simulink library "sm_car_lib"  (R2024a)
settings: Solver=VariableStepAuto  StartTime=0.0  StopTime=10.0  RelTol=1e-3
undefined symbols (not defined in the file or in its folder): acc_theta, accel_ramp_rate, circ_out, clr_upr, Control, hp1, hp2, hp3, hp_in_f_ua, hp_in_r_ua, hp_la_out, hp_ua_out, Init, Newton, opc_upr, radius_upr, Raphson, RDF_Rough_Road, rhs_hp, Scene, ShaftF, ShaftR, Vehicle, Visual, X, Y, Z
libraries: sm_lib x117, $bdroot x97, nesl_utility x36, simulink x17, fl_lib x6, sharedtransformsys x3, Brakes_Elements x2, Driver_Gamepad_Xbox x2, Multibody_Parts_Lib x2, sm_car_scene_track_mallory_park_obstacle x2, Testrig_4Post_Inputs x2, Aero_Coefficients x1
(part 7 of 7)

== system sm_car_lib/Environment/CarWorldConfig/Mechanism Configuration/Constant Gravity ==
  MechanismConfiguration : sm_lib/Utilities/Mechanism Configuration  UniformGravity=Constant  GravityVector=GravityVector  GravityVectorUnits=m/s^2  LinearizationDelta=0.001  JointModeTransitionNonlinearIterations=2
  C : PMIOPort  Side=Right
  connections:
  MechanismConfiguration/RConn1 -- C/RConn1

== system sm_car_lib/Environment/CarWorldConfig/Mechanism Configuration/Variable GravityXY ==
  Constant : Constant  Value=acc_theta
  Constant1 : Constant  Value=GravityVector(3)
  MechanismConfiguration : sm_lib/Utilities/Mechanism Configuration  UniformGravity=TimeVarying  GravityVector=[0 0 -9.80665]  GravityVectorUnits=m/s^2  LinearizationDelta=0.001  JointModeTransitionNonlinearIterations=2
  Mux : Mux  Inputs=3
  Product : Product
  Product1 : Product
  Ramp1 : simulink/Sources/Ramp  slope=accel_ramp_rate  start=2  InitialOutput=0
  Scope : Scope
  Simulink-PS Converter : nesl_utility/Simulink-PS Converter  PhysicalDomain=network_engine_domain  SubClassName=ps_input  LeftPortType=input  RightPortType=output  PseudoPeriodic=off  Frequencies=[]  NoiseDistribution=none  NoiseParameters=[]  Unit=m/s^2  AffineConversion=off  FilteringAndDerivatives=provide  SimscapeFilterOrder=1  InputFilterTimeConstant=0.001  UdotUserProvided=0
  Sin : Trigonometry
  Sin1 : Trigonometry  Operator=cos
  C : PMIOPort  Side=Right
  wires:
  Ramp1/1 -> Product/2, Product1/2, Scope/1  "accel_xy"
  Product1/1 -> Mux/1
  Constant1/1 -> Mux/3
  Sin/1 -> Product/1
  Mux/1 -> Simulink-PS Converter/1
  Sin1/1 -> Product1/1
  Constant/1 -> Sin/1, Sin1/1
  Product/1 -> Mux/2
  connections:
  MechanismConfiguration/LConn1 -- Simulink-PS Converter/RConn1
  MechanismConfiguration/RConn1 -- C/RConn1

== system sm_car_lib/Inputs/Control Bus/Torque Input/Torque Front ==
  Gain : Gain
  Rate Limiter : RateLimiter  RisingSlewLimit=300  FallingSlewLimit=-300  SampleTimeMode=inherited
  Step Height : Gain  Gain=torque_value
  Step Off : Step  Time=off_time  After=-1  SampleTime=0  ZeroCross=off
  Step On : Step  Time=on_time  SampleTime=0  ZeroCross=off
  Sum : Sum  Inputs=|++
  MMotorRDemand : Outport  VectorParamsAs1DForOutWhenUnconnected=off
  wires:
  Gain/1 -> MMotorRDemand/1  "MMotorRDemand"
  Step Off/1 -> Sum/2
  Sum/1 -> Step Height/1
  Step On/1 -> Sum/1
  Rate Limiter/1 -> Gain/1
  Step Height/1 -> Rate Limiter/1

== system sm_car_lib/Inputs/Control Bus/Torque Input/Torque Rear ==
  Gain : Gain
  Rate Limiter : RateLimiter  RisingSlewLimit=300  FallingSlewLimit=-300  SampleTimeMode=inherited
  Step Height : Gain  Gain=torque_value
  Step Off : Step  Time=off_time  After=-1  SampleTime=0  ZeroCross=off
  Step On : Step  Time=on_time  SampleTime=0  ZeroCross=off
  Sum : Sum  Inputs=|++
  MMotorRDemand : Outport  VectorParamsAs1DForOutWhenUnconnected=off
  wires:
  Step Height/1 -> Rate Limiter/1
  Rate Limiter/1 -> Gain/1
  Step On/1 -> Sum/1
  Sum/1 -> Step Height/1
  Step Off/1 -> Sum/2
  Gain/1 -> MMotorRDemand/1  "MMotorRDemand"

== system sm_car_lib/Inputs/Control Bus Axle3/Torque Input/Torque Front ==
  Gain : Gain
  Rate Limiter : RateLimiter  RisingSlewLimit=300  FallingSlewLimit=-300  SampleTimeMode=inherited
  Step Height : Gain  Gain=torque_value
  Step Off : Step  Time=off_time  After=-1  SampleTime=0  ZeroCross=off
  Step On : Step  Time=on_time  SampleTime=0  ZeroCross=off
  Sum : Sum  Inputs=|++
  MMotorRDemand : Outport  VectorParamsAs1DForOutWhenUnconnected=off
  wires:
  Step Height/1 -> Rate Limiter/1
  Rate Limiter/1 -> Gain/1
  Step On/1 -> Sum/1
  Sum/1 -> Step Height/1
  Step Off/1 -> Sum/2
  Gain/1 -> MMotorRDemand/1  "MMotorRDemand"

== system sm_car_lib/Inputs/Control Bus Axle3/Torque Input/Torque Rear ==
  Gain : Gain
  Rate Limiter : RateLimiter  RisingSlewLimit=300  FallingSlewLimit=-300  SampleTimeMode=inherited
  Step Height : Gain  Gain=torque_value
  Step Off : Step  Time=off_time  After=-1  SampleTime=0  ZeroCross=off
  Step On : Step  Time=on_time  SampleTime=0  ZeroCross=off
  Sum : Sum  Inputs=|++
  MMotorRDemand : Outport  VectorParamsAs1DForOutWhenUnconnected=off
  wires:
  Gain/1 -> MMotorRDemand/1  "MMotorRDemand"
  Step Off/1 -> Sum/2
  Sum/1 -> Step Height/1
  Step On/1 -> Sum/1
  Rate Limiter/1 -> Gain/1
  Step Height/1 -> Rate Limiter/1

== system sm_car_lib/Inputs/DrvBus/Torque Input/Torque Front ==
  Gain : Gain  Gain=rPedalValue
  Step Off : Step  Time=off_time  After=-1  SampleTime=0  ZeroCross=off
  Step On : Step  Time=on_time  SampleTime=0  ZeroCross=off
  Sum : Sum  Inputs=|++
  rAccelPedal : Outport  VectorParamsAs1DForOutWhenUnconnected=off
  wires:
  Sum/1 -> Gain/1
  Step Off/1 -> Sum/2
  Step On/1 -> Sum/1
  Gain/1 -> rAccelPedal/1  "rAccelPedal"

== system sm_car_lib/Outputs/VehBus/Brakes/Subsystem ==
  Bus Creator : BusCreator  Inputs=2
  Constant : Constant
  Constant1 : Constant
  Whl : Outport  VectorParamsAs1DForOutWhenUnconnected=off
  wires:
  Constant/1 -> Bus Creator/1  "trq"
  Bus Creator/1 -> Whl/1
  Constant1/1 -> Bus Creator/2  "p"

== system sm_car_lib/Outputs/VehBus/Subsystem/Aero ==
  Bus Creator : BusCreator  Inputs=2
  Constant1 : Constant
  Constant3 : Constant
  Aero : Outport  VectorParamsAs1DForOutWhenUnconnected=off
  wires:
  Constant3/1 -> Bus Creator/1  "Fx"
  Constant1/1 -> Bus Creator/2  "Fz"
  Bus Creator/1 -> Aero/1  "Aero"

== system sm_car_lib/Outputs/VehBus/Subsystem/Damper ==
  Bus Creator5 : BusCreator  Inputs=4
  Subsystem : Subsystem
  Subsystem1 : $bdroot/Outputs/VehBus/Subsystem/Damper/Subsystem  SystemSampleTime=-1  VariantActivationTime=update diagram  AllowFlexibleInterface=on  Latency=0  AutoFrameSizeCalculation=off
  Subsystem2 : $bdroot/Outputs/VehBus/Subsystem/Damper/Subsystem  SystemSampleTime=-1  VariantActivationTime=update diagram  AllowFlexibleInterface=on  Latency=0  AutoFrameSizeCalculation=off
  Subsystem3 : $bdroot/Outputs/VehBus/Subsystem/Damper/Subsystem  SystemSampleTime=-1  VariantActivationTime=update diagram  AllowFlexibleInterface=on  Latency=0  AutoFrameSizeCalculation=off
  Damper : Outport  VectorParamsAs1DForOutWhenUnconnected=off
  wires:
  Subsystem3/1 -> Bus Creator5/4  "R2"
  Subsystem1/1 -> Bus Creator5/2  "R1"
  Bus Creator5/1 -> Damper/1  "Damper"
  Subsystem2/1 -> Bus Creator5/3  "L2"
  Subsystem/1(out) -> Bus Creator5/1  "L1"

== system sm_car_lib/Outputs/VehBus/Subsystem/Source ==
  Bus Creator : BusCreator  Inputs=15
  Constant1 : Constant  Value=[1 1 1]
  Constant{2..5,7..15} (13 alike) : Constant
  Constant6 : Constant  Value=[1 1 1]
  Whl : Outport  VectorParamsAs1DForOutWhenUnconnected=off
  wires:
  Constant11/1 -> Bus Creator/3  "n"
  Constant12/1 -> Bus Creator/4  "Fx"
  Constant1/1 -> Bus Creator/2  "xyz"
  Constant6/1 -> Bus Creator/1  "qxyz"
  Bus Creator/1 -> Whl/1
  Constant2/1 -> Bus Creator/5  "Fy"
  Constant3/1 -> Bus Creator/6  "Fz"
  Constant4/1 -> Bus Creator/7  "Mx"
  Constant5/1 -> Bus Creator/8  "My"
  Constant7/1 -> Bus Creator/9  "Mz"
  Constant8/1 -> Bus Creator/10  "rSlip"
  Constant9/1 -> Bus Creator/11  "aSlip"
  Constant10/1 -> Bus Creator/12  "aCamber"
  Constant13/1 -> Bus Creator/13  "vx"
  Constant14/1 -> Bus Creator/14  "rMuX"
  Constant15/1 -> Bus Creator/15  "rMuY"

== system sm_car_lib/Outputs/VehBus/Subsystem/Spring ==
  Bus Creator5 : BusCreator  Inputs=4
  Source : Subsystem
  Subsystem1 : $bdroot/Outputs/VehBus/Subsystem/Spring/Source  SystemSampleTime=-1  VariantActivationTime=update diagram  AllowFlexibleInterface=on  Latency=0  AutoFrameSizeCalculation=off
  Subsystem2 : $bdroot/Outputs/VehBus/Subsystem/Spring/Source  SystemSampleTime=-1  VariantActivationTime=update diagram  AllowFlexibleInterface=on  Latency=0  AutoFrameSizeCalculation=off
  Subsystem3 : $bdroot/Outputs/VehBus/Subsystem/Spring/Source  SystemSampleTime=-1  VariantActivationTime=update diagram  AllowFlexibleInterface=on  Latency=0  AutoFrameSizeCalculation=off
  Spring : Outport  VectorParamsAs1DForOutWhenUnconnected=off
  wires:
  Bus Creator5/1 -> Spring/1  "Spring"
  Subsystem1/1 -> Bus Creator5/2  "R1"
  Subsystem2/1 -> Bus Creator5/3  "L2"
  Subsystem3/1 -> Bus Creator5/4  "R2"
  Source/1(out) -> Bus Creator5/1  "L1"

== system sm_car_lib/Sensors/Body Sensor/Roll Pitch/Calculate aPitch ==
  Roll Angle : Inport
  uvec : Inport  Port=2
  Asin : Trigonometry  Operator=asin
  Cos : Trigonometry  Operator=cos
  Divide : Product  Inputs=*/
  Divide1 : Product  Inputs=*/
  Selector : Selector  InputPortWidth=3  IndexOptions=Index vector (dialog)  Indices=[3]  OutputSizes=1
  magnitude : Fcn  Expr=sqrt(u(1)*u(1)+u(2)*u(2)+u(3)*u(3))
  Angle : Outport  VectorParamsAs1DForOutWhenUnconnected=off
  wires:
  Divide1/1 -> Asin/1
  uvec/1 -> magnitude/1, Selector/1
  magnitude/1 -> Divide1/2
  Selector/1 -> Divide/1
  Roll Angle/1 -> Cos/1
  Asin/1 -> Angle/1
  Divide/1 -> Divide1/1
  Cos/1 -> Divide/2

== system sm_car_lib/Sensors/Body Sensor/Roll Pitch/Calculate aRoll ==
  uvec : Inport
  Demux : Demux  Outputs=3
  Mux : Mux  Inputs=2
  Trigonometric Function1 : Trigonometry  Operator=atan2
  magnitude : Fcn  Expr=sqrt(u(1)*u(1)+u(2)*u(2))
  Angle : Outport  VectorParamsAs1DForOutWhenUnconnected=off
  wires:
  Demux/2 -> Mux/2
  magnitude/1 -> Trigonometric Function1/2
  Mux/1 -> magnitude/1
  Demux/3 -> Trigonometric Function1/1
  Trigonometric Function1/1 -> Angle/1
  uvec/1 -> Demux/1
  Demux/1 -> Mux/1

== system sm_car_lib/Utilities/Q to Z-Y-X Extrinsic/Subsystem/Subsystem ==
  In : Inport
  If : If  IfExpression=u1 > 1  ElseIfExpressions=u1 < -1
  If Action Subsystem : sharedtransformsys/Protect asincos input/If Action Subsystem  SystemSampleTime=-1  VariantActivationTime=update diagram  AllowFlexibleInterface=on  Latency=0  AutoFrameSizeCalculation=off
  If Action Subsystem1 : sharedtransformsys/Protect asincos input/If Action Subsystem1  SystemSampleTime=-1  VariantActivationTime=update diagram  AllowFlexibleInterface=on  Latency=0  AutoFrameSizeCalculation=off
  If Action Subsystem2 : sharedtransformsys/Protect asincos input/If Action Subsystem2  SystemSampleTime=-1  VariantActivationTime=update diagram  AllowFlexibleInterface=on  Latency=0  AutoFrameSizeCalculation=off
  Merge : Merge  Inputs=3
  Out : Outport  VectorParamsAs1DForOutWhenUnconnected=off
  wires:
  If Action Subsystem1/1 -> Merge/2
  If/1 -> If Action Subsystem/Action
  In/1 -> If/1, If Action Subsystem2/1
  If/3 -> If Action Subsystem2/Action
  If Action Subsystem2/1 -> Merge/3
  If/2 -> If Action Subsystem1/Action
  If Action Subsystem/1 -> Merge/1
  Merge/1 -> Out/1

== system sm_car_lib/Utilities/Q to Z-Y-X Extrinsic/Subsystem1/Subsystem ==
  In1 : Inport
  Demux : Demux
  Product{,1..3} (4 alike) : Product
  Sum : Sum  Inputs=4
  sqrt : Sqrt  AlgorithmType=Newton-Raphson
  Out1 : Outport  VectorParamsAs1DForOutWhenUnconnected=off
  wires:
  Sum/1 -> sqrt/1
  sqrt/1 -> Out1/1
  In1/1 -> Demux/1
  Product3/1 -> Sum/4
  Demux/2 -> Product1/1, Product1/2
  Demux/1 -> Product/1, Product/2
  Product2/1 -> Sum/3
  Product/1 -> Sum/1
  Demux/3 -> Product2/1, Product2/2
  Product1/1 -> Sum/2
  Demux/4 -> Product3/1, Product3/2

== system sm_car_lib/Control/Brake Control/ABS/Sensor/missing tooth ==
  <omega> : Inport
  <qxyz> : Inport  Port=2
  Constant : Constant  Value=2*pi
  Constant1 : Constant  Value=0.5
  Constant2 : Constant
  Product : Product
  Rem : Math  Operator=rem  SignedPower=on
  Scope : Scope  NumInputPorts=5
  Selector : Selector  InputPortWidth=3  IndexOptions=Index vector (dialog)  Indices=[2]  OutputSizes=1
  Subsystem : Subsystem  mask{int_limit_upper=25/48*2*pi, int_limit_lower=22/48*2*pi}
      mask prompts: int_limit_upper "Upper Limit"; int_limit_lower "Lower Limit"
      mask TypeOptions int_limit_upper: Upper Limit/Value
      mask TypeOptions int_limit_lower: Lower Limit/Value
  Switch : Switch  Criteria=u2 > Threshold  Threshold=0.5  SaturateOnIntegerOverflow=off  InputSameDT=off
  Out1 : Outport  VectorParamsAs1DForOutWhenUnconnected=off
  wires:
  <qxyz>/1 -> Scope/1, Selector/1
  Constant/1 -> Rem/2
  Rem/1 -> Scope/3, Subsystem/1(u)
  Selector/1 -> Scope/2, Rem/1
  Subsystem/1(y) -> Scope/4, Switch/2
  Switch/1 -> Scope/5, Product/2
  Constant1/1 -> Switch/1
  Constant2/1 -> Switch/3
  <omega>/1 -> Product/1
  Product/1 -> Out1/1

== system sm_car_lib/Outputs/VehBus/Subsystem/Damper/Subsystem ==
  Bus Creator : BusCreator  Inputs=4
  Constant{1..4} (4 alike) : Constant
  out : Outport  VectorParamsAs1DForOutWhenUnconnected=off
  wires:
  Constant2/1 -> Bus Creator/3  "xDamper"
  Bus Creator/1 -> out/1
  Constant3/1 -> Bus Creator/4  "vDamper"
  Constant1/1 -> Bus Creator/2  "FBumpstop"
  Constant4/1 -> Bus Creator/1  "FDamper"

== system sm_car_lib/Outputs/VehBus/Subsystem/Spring/Source ==
  Bus Creator : BusCreator  Inputs=2
  Constant1 : Constant
  Constant4 : Constant
  out : Outport  VectorParamsAs1DForOutWhenUnconnected=off
  wires:
  Constant1/1 -> Bus Creator/2  "FSpring"
  Constant4/1 -> Bus Creator/1  "xSpring"
  Bus Creator/1 -> out/1

== system sm_car_lib/Control/Brake Control/ABS/Sensor/missing tooth/Subsystem ==
  u : Inport
  AND : Logic  AllPortsSameDT=off  OutDataTypeStr=boolean
  FixPt Data Type Duplicate : DataTypeDuplicate  DisableCoverage=on  NumInputPorts=3
  Lower Limit : Constant  DisableCoverage=on  Value=int_limit_lower  OutDataTypeStr=Inherit: Inherit via back propagation
  Lower Test : RelationalOperator  DisableCoverage=on  Operator=<=  OutDataTypeStr=boolean  InputSameDT=off
  Upper Limit : Constant  DisableCoverage=on  Value=int_limit_upper  OutDataTypeStr=Inherit: Inherit via back propagation
  Upper Test : RelationalOperator  DisableCoverage=on  Operator=<=  OutDataTypeStr=boolean  InputSameDT=off
  y : Outport  VectorParamsAs1DForOutWhenUnconnected=off
  wires:
  Lower Limit/1 -> FixPt Data Type Duplicate/2, Lower Test/1
  Upper Limit/1 -> FixPt Data Type Duplicate/3, Upper Test/2
  u/1 -> Upper Test/1, Lower Test/2, FixPt Data Type Duplicate/1
  AND/1 -> y/1
  Upper Test/1 -> AND/2
  Lower Test/1 -> AND/1

== stateflow chart sm_car_lib/Control/Valve Control/Logic ==
  state Inactive
    entry:
    Mod_State = 1;
    Mod_Dur = 10;
  state Initial_Release
    entry:
    Mod_State = 2;
    Mod_Dur = 10;
  state Initial_Apply
    entry:
    Mod_State = 1;
    Mod_Dur = 6;
  state Release
    entry:
    Mod_State = 2;
    Mod_Dur = 6;
  state Apply
    entry:
    Mod_State = 1;
    Mod_Dur = 2;
  state Hold
    entry:
    Mod_State = 0;
    Mod_Dur = 6;
  (default) -> Inactive
  Apply -> Inactive [order 2] : [vSpdEst <0.1]
  Release -> Inactive [order 2] : [vSpdEst <0.1]
  Inactive -> Initial_Release : [Slip>0.5]
  Initial_Release -> Initial_Apply : [Slip<0.1]
  Release -> Initial_Apply [order 1] : [Slip <0.05]
  Initial_Apply -> Hold [order 2] : [Slip>0.1]
  Initial_Apply -> Apply [order 1] : [after(10,msec)]
  Hold -> Release [order 2] : [Slip > 0.25]
  Hold -> Apply [order 1] : [after(40,msec)]
  Apply -> Hold [order 1] : [Slip > 0.1]
  data: Slip input; Mod_State output; Mod_Dur output; vSpdEst input
